simulink model "Maxpid_fermeture_geometrique_2016a"  (R2016b)
settings: Solver=VariableStepAuto  StartTime=0.0  StopTime=10.0  RelTol=1e-3
PreLoadFcn:
  | addpath('Simscape')
model workspace (MATLAB code in the model file):
  | % Simscape(TM) Multibody(TM) version: 7.0
  | 
  | % This is a model data file derived from a Simscape Multibody Import XML file using the smimport function.
  | % The data in this file sets the block parameter values in an imported Simscape Multibody model.
  | % For more information on this file, see the smimport function help page in the Simscape Multibody documentation.
  | % You can modify numerical values, but avoid any other changes to this file.
  | % Do not add code to this file. Do not edit the physical units shown in comments.
  | 
  | %%%VariableName:smiData
  | 
  | 
  | %============= RigidTransform =============%
  | 
  | %Initialize the RigidTransform structure array by filling in null values.
  | smiData.RigidTransform(52).translation = [0.0 0.0 0.0];
  | smiData.RigidTransform(52).angle = 0.0;
  | smiData.RigidTransform(52).axis = [0.0 0.0 0.0];
  | smiData.RigidTransform(52).ID = '';
  | 
  | %Translation Method - Cartesian
  | %Rotation Method - Arbitrary Axis
  | smiData.RigidTransform(1).translation = [-10.000000000000057 1.9247813558290127e-14 5.0621138792892188e-15];  % mm
  | smiData.RigidTransform(1).angle = 2.0943951023931962;  % rad
  | smiData.RigidTransform(1).axis = [-0.57735026918962473 -0.57735026918962606 0.57735026918962651];
  | smiData.RigidTransform(1).ID = 'B[vis_ass-1:-:moteur_ass-1]';
  | 
  | %Translation Method - Cartesian
  | %Rotation Method - Arbitrary Axis
  | smiData.RigidTransform(2).translation = [200.00000000000006 0.0020410288675948296 4.1211478674085811e-13];  % mm
  | smiData.RigidTransform(2).angle = 2.0943951023931966;  % rad
  | smiData.RigidTransform(2).axis = [-0.57735026918962606 -0.57735026918962618 0.57735026918962506];
  | smiData.RigidTransform(2).ID = 'F[vis_ass-1:-:moteur_ass-1]';
  | 
  | %Translation Method - Cartesian
  | %Rotation Method - Arbitrary Axis
  | smiData.RigidTransform(3).translation = [79.999999999999986 1.1487735351088687e-14 12.999999999999844];  % mm
  | smiData.RigidTransform(3).angle = 1.6411050513807407e-15;  % rad
  | smiData.RigidTransform(3).axis = [0.99999999925342131 -3.864139429547283e-05 -3.1707293661675708e-20];
  | smiData.RigidTransform(3).ID = 'B[bras_ass-1:-:ecrou_ass-1]';
  | 
  | %Translation Method - Cartesian
  | %Rotation Method - Arbitrary Axis
  | smiData.RigidTransform(4).translation = [7.6827433304060833e-14 -3.4283687000424834e-13 15.979130371550594];  % mm
  | smiData.RigidTransform(4).angle = 1.3742753698359832e-14;  % rad
  | smiData.RigidTransform(4).axis = [0.99516609511328202 -0.098206125760982824 -6.7154932536581202e-16];
  | smiData.RigidTransform(4).ID = 'F[bras_ass-1:-:ecrou_ass-1]';
  | 
  | %Translation Method - Cartesian
  | %Rotation Method - Arbitrary Axis
  | smiData.RigidTransform(5).translation = [-10.000000000000057 1.9247813558290127e-14 5.0621138792892188e-15];  % mm
  | smiData.RigidTransform(5).angle = 2.0943951023931962;  % rad
  | smiData.RigidTransform(5).axis = [-0.57735026918962473 -0.57735026918962606 0.57735026918962651];
  | smiData.RigidTransform(5).ID = 'B[vis_ass-1:-:ecrou_ass-1]';
  | 
  | %Translation Method - Cartesian
  | %Rotation Method - Arbitrary Axis
  | smiData.RigidTransform(6).translation = [-30.000729304908297 -0.50000000000034284 5.9791303715506583];  % mm
  | smiData.RigidTransform(6).angle = 2.0943951023931957;  % rad
  | smiData.RigidTransform(6).axis = [0.57735026918962562 0.57735026918962584 0.57735026918962584];
  | smiData.RigidTransform(6).ID = 'F[vis_ass-1:-:ecrou_ass-1]';
  | 
  | %Translation Method - Cartesian
  | %Rotation Method - Arbitrary Axis
  | smiData.RigidTransform(7).translation = [1.4210854715202004e-14 -1.4210854715202004e-14 -46.499999999999986];  % mm
  | smiData.RigidTransform(7).angle = 3.1401849173675503e-16;  % rad
  | smiData.RigidTransform(7).axis = [-0.70710678118654746 -0.70710678118654746 7.8504622934188746e-17];
  | smiData.RigidTransform(7).ID = 'B[bras_ass-1:-:bati_ass-1]';
  | 
  | %Translation Method - Cartesian
  | %Rotation Method - Arbitrary Axis
  | smiData.RigidTransform(8).translation = [1.4210854715202016e-14 -7.1054273576010019e-15 -48.499999999999993];  % mm
  | smiData.RigidTransform(8).angle = 4.9650683064945482e-16;  % rad
  | smiData.RigidTransform(8).axis = [-0.89442719099991519 -0.44721359549995904 9.9301366129891115e-17];
  | smiData.RigidTransform(8).ID = 'F[bras_ass-1:-:bati_ass-1]';
  | 
  | %Translation Method - Cartesian
  | %Rotation Method - Arbitrary Axis
  | smiData.RigidTransform(9).translation = [0 0 0];  % mm
  | smiData.RigidTransform(9).angle = 2.0943951023931953;  % rad
  | smiData.RigidTransform(9).axis = [-0.57735026918962584 -0.57735026918962584 -0.57735026918962584];
  | smiData.RigidTransform(9).ID = 'B[bati_ass-1:-:]';
  | 
  | %Translation Method - Cartesian
  | %Rotation Method - Arbitrary Axis
  | smiData.RigidTransform(10).translation = [0 0 0];  % mm
  | smiData.RigidTransform(10).angle = 1.5707963267948966;  % rad
  | smiData.RigidTransform(10).axis = [7.8504622934188758e-17 7.8504622934188758e-17 -1];
  | smiData.RigidTransform(10).ID = 'F[bati_ass-1:-:]';
  | 
  | %Translation Method - Cartesian
  | %Rotation Method - Arbitrary Axis
  | smiData.RigidTransform(11).translation = [-70 80 -33];  % mm
  | smiData.RigidTransform(11).angle = 0;  % rad
  | smiData.RigidTransform(11).axis = [0 0 0];
  | smiData.RigidTransform(11).ID = 'B[bati_ass-1:-:moteur_ass-1]';
  | 
  | %Translation Method - Cartesian
  | %Rotation Method - Arbitrary Axis
  | smiData.RigidTransform(12).translation = [8.5265128291212022e-14 1.7053025658242404e-13 -33.999999999999822];  % mm
  | smiData.RigidTransform(12).angle = 5.4944824200518475e-15;  % rad
  | smiData.RigidTransform(12).axis = [0.96259366809221403 -0.27094912834105328 -7.1651873630488301e-16];
  | smiData.RigidTransform(12).ID = 'F[bati_ass-1:-:moteur_ass-1]';
  | 
  | %Translation Method - Cartesian
  | %Rotation Method - Arbitrary Axis
  | smiData.RigidTransform(13).translation = [90.999999999999744 0 -33.000000000000036];  % mm
  | smiData.RigidTransform(13).angle = 3.1415926535897865;  % rad
  | smiData.RigidTransform(13).axis = [-0 -1 -0];
  | smiData.RigidTransform(13).ID = 'AssemblyGround[bras_ass-1:VisChcM4-2]';
  | 
  | %Translation Method - Cartesian
  | %Rotation Method - Arbitrary Axis
  | smiData.RigidTransform(14).translation = [79.999999999999346 8.4654505627668196e-13 -19.999999999997431];  % mm
  | smiData.RigidTransform(14).angle = 0.092778004913466591;  % rad
  | smiData.RigidTransform(14).axis = [3.4812448211815589e-13 -1.4459260087237306e-14 -1];
  | smiData.RigidTransform(14).ID = 'AssemblyGround[bras_ass-1:BagueIna12-1]';
  | 
  | %Translation Method - Cartesian
  | %Rotation Method - Arbitrary Axis
  | smiData.RigidTransform(15).translation = [79.999999999999986 0 19.999999999999844];  % mm
  | smiData.RigidTransform(15).angle = 3.1415926535897918;  % rad
  | smiData.RigidTransform(15).axis = [-0.99892422316352036 0.046372366525306442 3.8019289262458494e-17];
  | smiData.RigidTransform(15).ID = 'AssemblyGround[bras_ass-1:BagueIna12-2]';
  | 
  | %Translation Method - Cartesian
  | %Rotation Method - Arbitrary Axis
  | smiData.RigidTransform(16).translation = [0 0 47.499999999999972];  % mm
  | smiData.RigidTransform(16).angle = 2.0943951023931953;  % rad
  | smiData.RigidTransform(16).axis = [0.57735026918962573 -0.57735026918962573 0.57735026918962584];
  | smiData.RigidTransform(16).ID = 'AssemblyGround[bras_ass-1:AxeBras-1]';
  | 
  | %Translation Method - Cartesian
  | %Rotation Method - Arbitrary Axis
  | smiData.RigidTransform(17).translation = [100.50000000000018 121.50000000000016 27.999999999999993];  % mm
  | smiData.RigidTransform(17).angle = 1.5707963267948981;  % rad
  | smiData.RigidTransform(17).axis = [-0 -0 -1];
  | smiData.RigidTransform(17).ID = 'AssemblyGround[bras_ass-1:Bras-1]';
  | 
  | %Translation Method - Cartesian
  | %Rotation Method - Arbitrary Axis
  | smiData.RigidTransform(18).translation = [294.00000000000006 0 0];  % mm
  | smiData.RigidTransform(18).angle = 1.5707963267948966;  % rad
  | smiData.RigidTransform(18).axis = [0 0 -1];
  | smiData.RigidTransform(18).ID = 'AssemblyGround[bras_ass-1:Poids-3]';
  | 
  | %Translation Method - Cartesian
  | %Rotation Method - Arbitrary Axis
  | smiData.RigidTransform(19).translation = [282 0 0];  % mm
  | smiData.RigidTransform(19).angle = 1.5707963267948966;  % rad
  | smiData.RigidTransform(19).axis = [0 0 -1];
  | smiData.RigidTransform(19).ID = 'AssemblyGround[bras_ass-1:Poids-1]';
  | 
  | %Translation Method - Cartesian
  | %Rotation Method - Arbitrary Axis
  | smiData.RigidTransform(20).translation = [252.00000000000011 0 0];  % mm
  | smiData.RigidTransform(20).angle = 1.5744482311252364;  % rad
  | smiData.RigidTransform(20).axis = [-0.060320878582140823 -0.060320878582140816 -0.99635474767482157];
  | smiData.RigidTransform(20).ID = 'AssemblyGround[bras_ass-1:EcrouSerragePoids-2]';
  | 
  | %Translation Method - Cartesian
  | %Rotation Method - Arbitrary Axis
  | smiData.RigidTransform(21).translation = [91.000000000000028 0 32.999999999999993];  % mm
  | smiData.RigidTransform(21).angle = 0;  % rad
  | smiData.RigidTransform(21).axis = [0 0 0];
  | smiData.RigidTransform(21).ID = 'AssemblyGround[bras_ass-1:VisChcM4-1]';
  | 
  | %Translation Method - Cartesian
  | %Rotation Method - Arbitrary Axis
  | smiData.RigidTransform(22).translation = [80.000000000000028 0 29.999999999999982];  % mm
  | smiData.RigidTransform(22).angle = 3.1415926535897931;  % rad
  | smiData.RigidTransform(22).axis = [-0.70710678118654791 -0.70710678118654713 -3.9695354913923758e-17];
  | smiData.RigidTransform(22).ID = 'AssemblyGround[bras_ass-1:AxeArticulation-2]';
  | 
  | %Translation Method - Cartesian
  | %Rotation Method - Arbitrary Axis
  | smiData.RigidTransform(23).translation = [80.000000000000014 0 -29.999999999999989];  % mm
  | smiData.RigidTransform(23).angle = 1.5707963267948977;  % rad
  | smiData.RigidTransform(23).axis = [-0 -0 -1];
  | smiData.RigidTransform(23).ID = 'AssemblyGround[bras_ass-1:AxeArticulation-1]';
  | 
  | %Translation Method - Cartesian
  | %Rotation Method - Arbitrary Axis
  | smiData.RigidTransform(24).translation = [258.00000000000006 0 0];  % mm
  | smiData.RigidTransform(24).angle = 1.5708826466989811;  % rad
  | smiData.RigidTransform(24).axis = [-0.009290449585176894 -0.0092904495851768906 -0.999913683821264];
  | smiData.RigidTransform(24).ID = 'AssemblyGround[bras_ass-1:EcrouSerragePoids-1]';
  | 
  | %Translation Method - Cartesian
  | %Rotation Method - Arbitrary Axis
  | smiData.RigidTransform(25).translation = [237.00000000000009 3.4197923590601689 2.3580168307901075];  % mm
  | smiData.RigidTransform(25).angle = 2.718034541017071;  % rad
  | smiData.RigidTransform(25).axis = [-0.69056994469318977 -0.69056994469318989 -0.21500303014815719];
  | smiData.RigidTransform(25).ID = 'AssemblyGround[bras_ass-1:AxePoids-1]';
  | 
  | %Translation Method - Cartesian
  | %Rotation Method - Arbitrary Axis
  | smiData.RigidTransform(26).translation = [294.00000000000011 0 0];  % mm
  | smiData.RigidTransform(26).angle = 1.5987068466520886;  % rad
  | smiData.RigidTransform(26).axis = [0.16477027986751258 -0.16477027986751264 0.97247185550264792];
  | smiData.RigidTransform(26).ID = 'AssemblyGround[bras_ass-1:AxeRessort-1]';
  | 
  | %Translation Method - Cartesian
  | %Rotation Method - Arbitrary Axis
  | smiData.RigidTransform(27).translation = [270 0 0];  % mm
  | smiData.RigidTransform(27).angle = 1.5707963267948966;  % rad
  | smiData.RigidTransform(27).axis = [0 0 -1];
  | smiData.RigidTransform(27).ID = 'AssemblyGround[bras_ass-1:Poids-2]';
  | 
  | %Translation Method - Cartesian
  | %Rotation Method - Arbitrary Axis
  | smiData.RigidTransform(28).translation = [-200.00000000000011 0 0];  % mm
  | smiData.RigidTransform(28).angle = 1.6033476988916029;  % rad
  | smiData.RigidTransform(28).axis = [-0.17753814395804177 0.17753814395804177 0.96796715588901427];
  | smiData.RigidTransform(28).ID = 'AssemblyGround[vis_ass-1:EcrouM6-1]';
  | 
  | %Translation Method - Cartesian
  | %Rotation Method - Arbitrary Axis
  | smiData.RigidTransform(29).translation = [-176.00000000000009 0 0];  % mm
  | smiData.RigidTransform(29).angle = 0.51434614493842068;  % rad
  | smiData.RigidTransform(29).axis = [1 0 2.3568855398281085e-16];
  | smiData.RigidTransform(29).ID = 'AssemblyGround[vis_ass-1:VisBille-1]';
  | 
  | %Translation Method - Cartesian
  | %Rotation Method - Arbitrary Axis
  | smiData.RigidTransform(30).translation = [-10.000000000000009 0 0];  % mm
  | smiData.RigidTransform(30).angle = 0.94247779607696236;  % rad
  | smiData.RigidTransform(30).axis = [1 1.9209682992159078e-15 1.5599933518283066e-15];
  | smiData.RigidTransform(30).ID = 'AssemblyGround[vis_ass-1:RondelleVisBille-1]';
  | 
  | %Translation Method - Cartesian
  | %Rotation Method - Arbitrary Axis
  | smiData.RigidTransform(31).translation = [-207.00000000000014 0 0];  % mm
  | smiData.RigidTransform(31).angle = 1.2080018604776608;  % rad
  | smiData.RigidTransform(31).axis = [1 -8.9064014692544017e-17 0];
  | smiData.RigidTransform(31).ID = 'AssemblyGround[vis_ass-1:Accouplement-1]';
  | 
  | %Translation Method - Cartesian
  | %Rotation Method - Arbitrary Axis
  | smiData.RigidTransform(32).translation = [-195.00000000000017 0 0];  % mm
  | smiData.RigidTransform(32).angle = 2.8566332216390737;  % rad
  | smiData.RigidTransform(32).axis = [-0.69979339697627563 -0.14345174483710449 0.69979339697627541];
  | smiData.RigidTransform(32).ID = 'AssemblyGround[vis_ass-1:RondelleM6-1]';
  | 
  | %Translation Method - Cartesian
  | %Rotation Method - Arbitrary Axis
  | smiData.RigidTransform(33).translation = [-249.00000000000011 0 0];  % mm
  | smiData.RigidTransform(33).angle = 0.61326057885890328;  % rad
  | smiData.RigidTransform(33).axis = [1 -4.9895816407432893e-17 -5.3048086412437212e-16];
  | smiData.RigidTransform(33).ID = 'AssemblyGround[vis_ass-1:RotorMoteur-1]';
  | 
  | %Translation Method - Cartesian
  | %Rotation Method - Arbitrary Axis
  | smiData.RigidTransform(34).translation = [-179.00000000000006 0 0];  % mm
  | smiData.RigidTransform(34).angle = 0.072273946411088433;  % rad
  | smiData.RigidTransform(34).axis = [1 0 0];
  | smiData.RigidTransform(34).ID = 'AssemblyGround[vis_ass-1:BagueVisBille-1]';
  | 
  | %Translation Method - Cartesian
  | %Rotation Method - Arbitrary Axis
  | smiData.RigidTransform(35).translation = [-3.0000000000000444 0 0];  % mm
  | smiData.RigidTransform(35).angle = 0.82843866056758242;  % rad
  | smiData.RigidTransform(35).axis = [1 -1.1299952875043414e-16 7.5333019166956099e-17];
  | smiData.RigidTransform(35).ID = 'AssemblyGround[vis_ass-1:VisFhcM6-1]';
  | 
  | %Translation Method - Cartesian
  | %Rotation Method - Arbitrary Axis
  | smiData.RigidTransform(36).translation = [-193.00000000000011 0 0];  % mm
  | smiData.RigidTransform(36).angle = 1.136496024515387;  % rad
  | smiData.RigidTransform(36).axis = [-1 -1.1885914893422454e-16 1.223838459411135e-16];
  | smiData.RigidTransform(36).ID = 'AssemblyGround[vis_ass-1:BagueIntRoulement-1]';
  | 
  | %Translation Method - Cartesian
  | %Rotation Method - Arbitrary Axis
  | smiData.RigidTransform(37).translation = [-30 0.0020410288673958221 -21.499999999999613];  % mm
  | smiData.RigidTransform(37).angle = 1.6664335535985522;  % rad
  | smiData.RigidTransform(37).axis = [-0.29524180884432899 -0.90866085456602452 0.29524180884432827];
  | smiData.RigidTransform(37).ID = 'AssemblyGround[moteur_ass-1:VisChcM4-2]';
  | 
  | %Translation Method - Cartesian
  | %Rotation Method - Arbitrary Axis
  | smiData.RigidTransform(38).translation = [19.999999999999989 0.0020410288674443944 0];  % mm
  | smiData.RigidTransform(38).angle = 0.62831853071796473;  % rad
  | smiData.RigidTransform(38).axis = [-1 -2.8889459081957584e-15 -1.127557849593959e-15];
  | smiData.RigidTransform(38).ID = 'AssemblyGround[moteur_ass-1:SupprotVisBille-1]';
  | 
  | %Translation Method - Cartesian
  | %Rotation Method - Arbitrary Axis
  | smiData.RigidTransform(39).translation = [20.000000000000018 0.0020410288674374555 0];  % mm
  | smiData.RigidTransform(39).angle = 0.65731557306984645;  % rad
  | smiData.RigidTransform(39).axis = [1 -2.9269271194518664e-15 6.3474248646130781e-16];
  | smiData.RigidTransform(39).ID = 'AssemblyGround[moteur_ass-1:BagueExtRoulement-1]';
  | 
  | %Translation Method - Cartesian
  | %Rotation Method - Arbitrary Axis
  | smiData.RigidTransform(40).translation = [34.000000000000014 0.0020410288674374555 0];  % mm
  | smiData.RigidTransform(40).angle = 0.032120796998705951;  % rad
  | smiData.RigidTransform(40).axis = [1 0 0];
  | smiData.RigidTransform(40).ID = 'AssemblyGround[moteur_ass-1:EcrouSupportVisBille-1]';
  | 
  | %Translation Method - Cartesian
  | %Rotation Method - Arbitrary Axis
  | smiData.RigidTransform(41).translation = [-30.000000000000028 0.0020410288675068444 21.499999999999595];  % mm
  | smiData.RigidTransform(41).angle = 1.6664335535985522;  % rad
  | smiData.RigidTransform(41).axis = [-0.29524180884432899 -0.90866085456602452 0.29524180884432827];
  | smiData.RigidTransform(41).ID = 'AssemblyGround[moteur_ass-1:VisChcM4-1]';
  | 
  | %Translation Method - Cartesian
  | %Rotation Method - Arbitrary Axis
  | smiData.RigidTransform(42).translation = [-26.999999999999996 0.0020410288674513333 0];  % mm
  | smiData.RigidTransform(42).angle = 2.1991148575128614;  % rad
  | smiData.RigidTransform(42).axis = [-1 -4.8071886820195462e-16 -9.4749987733508383e-16];
  | smiData.RigidTransform(42).ID = 'AssemblyGround[moteur_ass-1:BrideMoteur-1]';
  | 
  | %Translation Method - Cartesian
  | %Rotation Method - Arbitrary Axis
  | smiData.RigidTransform(43).translation = [-31 0.0020410288674513333 0];  % mm
  | smiData.RigidTransform(43).angle = 0.050793545886475028;  % rad
  | smiData.RigidTransform(43).axis = [-1 -3.7517109526216934e-14 -1.4996924802690354e-15];
  | smiData.RigidTransform(43).ID = 'AssemblyGround[moteur_ass-1:StatorMoteur-1]';
  | 
  | %Translation Method - Cartesian
  | %Rotation Method - Arbitrary Axis
  | smiData.RigidTransform(44).translation = [-70.000000000000284 68.999999999999972 -35.999999999999467];  % mm
  | smiData.RigidTransform(44).angle = 3.1415926535897865;  % rad
  | smiData.RigidTransform(44).axis = [-0 -1 -0];
  | smiData.RigidTransform(44).ID = 'AssemblyGround[bati_ass-1:VisChcM4-2]';
  | 
  | %Translation Method - Cartesian
  | %Rotation Method - Arbitrary Axis
  | smiData.RigidTransform(45).translation = [0 0 46.000000000000085];  % mm
  | smiData.RigidTransform(45).angle = 3.1415926535897865;  % rad
  | smiData.RigidTransform(45).axis = [-1 -0 -0];
  | smiData.RigidTransform(45).ID = 'AssemblyGround[bati_ass-1:BagueIna30-2]';
  | 
  | %Translation Method - Cartesian
  | %Rotation Method - Arbitrary Axis
  | smiData.RigidTransform(46).translation = [0 0 -46];  % mm
  | smiData.RigidTransform(46).angle = 0;  % rad
  | smiData.RigidTransform(46).axis = [0 0 0];
  | smiData.RigidTransform(46).ID = 'AssemblyGround[bati_ass-1:BagueIna30-1]';
  | 
  | %Translation Method - Cartesian
  | %Rotation Method - Arbitrary Axis
  | smiData.RigidTransform(47).translation = [-69.999999999999986 79.999999999999972 33];  % mm
  | smiData.RigidTransform(47).angle = 3.1415926535897931;  % rad
  | smiData.RigidTransform(47).axis = [-1 -0 -0];
  | smiData.RigidTransform(47).ID = 'AssemblyGround[bati_ass-1:AxeArticulation-1]';
  | 
  | %Translation Method - Cartesian
  | %Rotation Method - Arbitrary Axis
  | smiData.RigidTransform(48).translation = [-70 80 -33];  % mm
  | smiData.RigidTransform(48).angle = 3.1415926535897931;  % rad
  | smiData.RigidTransform(48).axis = [0 0 1];
  | smiData.RigidTransform(48).ID = 'AssemblyGround[bati_ass-1:AxeArticulation-2]';
  | 
  | %Translation Method - Cartesian
  | %Rotation Method - Arbitrary Axis
  | smiData.RigidTransform(49).translation = [0 0 0];  % mm
  | smiData.RigidTransform(49).angle = 0;  % rad
  | smiData.RigidTransform(49).axis = [0 0 0];
  | smiData.RigidTransform(49).ID = 'AssemblyGround[bati_ass-1:Chaise-1]';
  | 
  | %Translation Method - Cartesian
  | %Rotation Method - Arbitrary Axis
  | smiData.RigidTransform(50).translation = [-70.000000000000014 69 36.000000000000007];  % mm
  | smiData.RigidTransform(50).angle = 0;  % rad
  | smiData.RigidTransform(50).axis = [0 0 0];
  | smiData.RigidTransform(50).ID = 'AssemblyGround[bati_ass-1:VisChcM4-1]';
  | 
  | %Translation Method - Cartesian
  | %Rotation Method - Arbitrary Axis
  | smiData.RigidTransform(51).translation = [40.125000000000036 16.792738254764792 -6.5847793962006174];  % mm
  | smiData.RigidTransform(51).angle = 0.62831853071794164;  % rad
  | smiData.RigidTransform(51).axis = [-1 0 0];
  | smiData.RigidTransform(51).ID = 'AssemblyGround[ecrou_ass-1:SupportEcrouBille-1]';
  | 
  | %Translation Method - Cartesian
  | %Rotation Method - Arbitrary Axis
  | smiData.RigidTransform(52).translation = [7.0000000000000338 -0.49999999999993106 5.9791303715507071];  % mm
  | smiData.RigidTransform(52).angle = 1.9713451234477288;  % rad
  | smiData.RigidTransform(52).axis = [0.52965656527971039 0.66251629845023408 0.52965656527971061];
  | smiData.RigidTransform(52).ID = 'AssemblyGround[ecrou_ass-1:EcrouBille-1]';
  | 
  | 
  | %============= Solid =============%
  | %Center of Mass (CoM) %Moments of Inertia (MoI) %Product of Inertia (PoI)
  | 
  | %Initialize the Solid structure array by filling in null values.
  | smiData.Solid(27).mass = 0.0;
  | smiData.Solid(27).CoM = [0.0 0.0 0.0];
  | smiData.Solid(27).MoI = [0.0 0.0 0.0];
  | smiData.Solid(27).PoI = [0.0 0.0 0.0];
  | smiData.Solid(27).color = [0.0 0.0 0.0];
  | smiData.Solid(27).opacity = 0.0;
  | smiData.Solid(27).ID = '';
  | 
  | %Inertia Type - Custom
  | %Visual Properties - Simple
  | smiData.Solid(1).mass = 1.913087125687861e-14;  % kg
  | smiData.Solid(1).CoM = [0.00017482716988745047 3.2099175360591674e-05 -1.3211998133732603];  % mm
  | smiData.Solid(1).MoI = [0 0 0];  % kg*mm^2
  | smiData.Solid(1).PoI = [0 0 0];  % kg*mm^2
  | smiData.Solid(1).color = [0.792156862745098 0.81960784313725488 0.93333333333333335];
  | smiData.Solid(1).opacity = 1;
  | smiData.Solid(1).ID = 'VisChcM4*:*Defaut';
  | 
  | %Inertia Type - Custom
  | %Visual Properties - Simple
  | smiData.Solid(2).mass = 4.8694686130641791e-14;  % kg
  | smiData.Solid(2).CoM = [0 0 1.848387096774194];  % mm
  | smiData.Solid(2).MoI = [0 0 0];  % kg*mm^2
  | smiData.Solid(2).PoI = [0 0 0];  % kg*mm^2
  | smiData.Solid(2).color = [1 0 0];
  | smiData.Solid(2).opacity = 1;
  | smiData.Solid(2).ID = 'BagueIna12*:*Defaut';
  | 
  | %Inertia Type - Custom
  | %Visual Properties - Simple
  | smiData.Solid(3).mass = 6.5992676097002718e-12;  % kg
  | smiData.Solid(3).CoM = [-48.219059130186579 0 0];  % mm
  | smiData.Solid(3).MoI = [7.4534196241053467e-10 5.1914505440532212e-09 5.1839580222850838e-09];  % kg*mm^2
  | smiData.Solid(3).PoI = [0 0 0];  % kg*mm^2
  | smiData.Solid(3).color = [1 0 0];
  | smiData.Solid(3).opacity = 1;
  | smiData.Solid(3).ID = 'AxeBras*:*Defaut';
  | 
  | %Inertia Type - Custom
  | %Visual Properties - Simple
  | smiData.Solid(4).mass = 1.1966905700493424e-11;  % kg
  | smiData.Solid(4).CoM = [121.52268202090545 -4.969129514901149 -27.999999999999556];  % mm
  | smiData.Solid(4).MoI = [7.7814080987725223e-08 6.582300775495296e-09 7.3498007295449486e-08];  % kg*mm^2
  | smiData.Solid(4).PoI = [0 0 0];  % kg*mm^2
  | smiData.Solid(4).color = [1 0 0];
  | smiData.Solid(4).opacity = 1;
  | smiData.Solid(4).ID = 'Bras*:*Defaut';
  | 
  | %Inertia Type - Custom
  | %Visual Properties - Simple
  | smiData.Solid(5).mass = 0.64789884834471512;  % kg
  | smiData.Solid(5).CoM = [-2.0536539050800404 -5.9999999999999627 0];  % mm
  | smiData.Solid(5).MoI = [448.87025526927192 835.42692079456913 402.10623788557024];  % kg*mm^2
  | smiData.Solid(5).PoI = [0 0 0];  % kg*mm^2
  | smiData.Solid(5).color = [1 0 0];
  | smiData.Solid(5).opacity = 1;
  | smiData.Solid(5).ID = 'Poids*:*Defaut';
  | 
  | %Inertia Type - Custom
  | %Visual Properties - Simple
  | smiData.Solid(6).mass = 1.1915826288096166e-13;  % kg
  | smiData.Solid(6).CoM = [3.6591475952249857e-05 -2.9997024398795644 2.6109734489883295e-05];  % mm
  | smiData.Solid(6).MoI = [0 0 0];  % kg*mm^2
  | smiData.Solid(6).PoI = [0 0 0];  % kg*mm^2
  | smiData.Solid(6).color = [1 0 0];
  | smiData.Solid(6).opacity = 1;
  | smiData.Solid(6).ID = 'EcrouSerragePoids*:*Defaut';
  | 
  | %Inertia Type - Custom
  | %Visual Properties - Simple
  | smiData.Solid(7).mass = 3.6367861956118845e-13;  % kg
  | smiData.Solid(7).CoM = [0 -0.11402656300615598 2.1307319223985894];  % mm
  | smiData.Solid(7).MoI = [0 0 0];  % kg*mm^2
  | smiData.Solid(7).PoI = [0 0 0];  % kg*mm^2
  | smiData.Solid(7).color = [0.792156862745098 0.81960784313725488 0.93333333333333335];
  | smiData.Solid(7).opacity = 1;
  | smiData.Solid(7).ID = 'AxeArticulation*:*Defaut';
  | 
  | %Inertia Type - Custom
  | %Visual Properties - Simple
  | smiData.Solid(8).mass = 1.2840039937491999e-12;  % kg
  | smiData.Solid(8).CoM = [-4.1541055520205505 9.4534863101010309 -2.6439442480407891e-06];  % mm
  | smiData.Solid(8).MoI = [1.2381504618383058e-09 0 1.238157782687606e-09];  % kg*mm^2
  | smiData.Solid(8).PoI = [0 0 0];  % kg*mm^2
  | smiData.Solid(8).color = [1 0 0];
  | smiData.Solid(8).opacity = 1;
  | smiData.Solid(8).ID = 'AxePoids*:*Defaut';
  | 
  | %Inertia Type - Custom
  | %Visual Properties - Simple
  | smiData.Solid(9).mass = 3.3431781821951382e-13;  % kg
  | smiData.Solid(9).CoM = [0 -8.3913860610806577 0];  % mm
  | smiData.Solid(9).MoI = [0 0 0];  % kg*mm^2
  | smiData.Solid(9).PoI = [0 0 0];  % kg*mm^2
  | smiData.Solid(9).color = [1 0 0];
  | smiData.Solid(9).opacity = 1;
  | smiData.Solid(9).ID = 'AxeRessort*:*Defaut';
  | 
  | %Inertia Type - Custom
  | %Visual Properties - Simple
  | smiData.Solid(10).mass = 3.2436540679646126e-14;  % kg
  | smiData.Solid(10).CoM = [6.6017426300604492e-05 -2.5001780719836924 0.00011392574116365407];  % mm
  | smiData.Solid(10).MoI = [0 0 0];  % kg*mm^2
  | smiData.Solid(10).PoI = [0 0 0];  % kg*mm^2
  | smiData.Solid(10).color = [0.75294117647058822 1 0.75294117647058822];
  | smiData.Solid(10).opacity = 1;
  | smiData.Solid(10).ID = 'EcrouM6*:*Defaut';
  | 
  | %Inertia Type - Custom
  | %Visual Properties - Simple
  | smiData.Solid(11).mass = 1.9275110826406196e-12;  % kg
  | smiData.Solid(11).CoM = [75.753758887885439 0 0];  % mm
  | smiData.Solid(11).MoI = [0 4.9885760188161509e-09 4.9885760188161509e-09];  % kg*mm^2
  | smiData.Solid(11).PoI = [0 0 0];  % kg*mm^2
  | smiData.Solid(11).color = [0.75294117647058822 1 0.75294117647058822];
  | smiData.Solid(11).opacity = 1;
  | smiData.Solid(11).ID = 'VisBille*:*Defaut';
  | 
  | %Inertia Type - Custom
  | %Visual Properties - Simple
  | smiData.Solid(12).mass = 1.2036446851756366e-12;  % kg
  | smiData.Solid(12).CoM = [4.9618277776521449 0.0099812415306071399 -0.013780904347995832];  % mm
  | smiData.Solid(12).MoI = [0 0 0];  % kg*mm^2
  | smiData.Solid(12).PoI = [0 0 0];  % kg*mm^2
  | smiData.Solid(12).color = [0.75294117647058822 1 0.75294117647058822];
  | smiData.Solid(12).opacity = 1;
  | smiData.Solid(12).ID = 'RondelleVisBille*:*Defaut';
  | 
  | %Inertia Type - Custom
  | %Visual Properties - Simple
  | smiData.Solid(13).mass = 5.6096059033133564e-13;  % kg
  | smiData.Solid(13).CoM = [-10.914959484771275 -0.0013517034619366178 0.0015391063193635405];  % mm
  | smiData.Solid(13).MoI = [0 0 0];  % kg*mm^2
  | smiData.Solid(13).PoI = [0 0 0];  % kg*mm^2
  | smiData.Solid(13).color = [0.75294117647058822 1 0.75294117647058822];
  | smiData.Solid(13).opacity = 1;
  | smiData.Solid(13).ID = 'Accouplement*:*Defaut';
  | 
  | %Inertia Type - Custom
  | %Visual Properties - Simple
  | smiData.Solid(14).mass = 2.5132741228718347e-14;  % kg
  | smiData.Solid(14).CoM = [0 0 -1.0000000000000002];  % mm
  | smiData.Solid(14).MoI = [0 0 0];  % kg*mm^2
  | smiData.Solid(14).PoI = [0 0 0];  % kg*mm^2
  | smiData.Solid(14).color = [0.75294117647058822 1 0.75294117647058822];
  | smiData.Solid(14).opacity = 1;
  | smiData.Solid(14).ID = 'RondelleM6*:*Defaut';
  | 
  | %Inertia Type - Custom
  | %Visual Properties - Simple
  | smiData.Solid(15).mass = 1.834794829451559e-12;  % kg
  | smiData.Solid(15).CoM = [-26.298256378060618 0 0];  % mm
  | smiData.Solid(15).MoI = [0 6.3221197317200813e-10 6.3221197317200813e-10];  % kg*mm^2
  | smiData.Solid(15).PoI = [0 0 0];  % kg*mm^2
  | smiData.Solid(15).color = [0.75294117647058822 1 0.75294117647058822];
  | smiData.Solid(15).opacity = 1;
  | smiData.Solid(15).ID = 'RotorMoteur*:*Defaut';
  | 
  | %Inertia Type - Custom
  | %Visual Properties - Simple
  | smiData.Solid(16).mass = 1.0814932709982914e-13;  % kg
  | smiData.Solid(16).CoM = [-3.2639947954490749 0 0];  % mm
  | smiData.Solid(16).MoI = [0 0 0];  % kg*mm^2
  | smiData.Solid(16).PoI = [0 0 0];  % kg*mm^2
  | smiData.Solid(16).color = [0.75294117647058822 1 0.75294117647058822];
  | smiData.Solid(16).opacity = 1;
  | smiData.Solid(16).ID = 'BagueVisBille*:*Defaut';
  | 
  | %Inertia Type - Custom
  | %Visual Properties - Simple
  | smiData.Solid(17).mass = 7.9381889668023803e-14;  % kg
  | smiData.Solid(17).CoM = [-8.1180211458661269 0 0];  % mm
  | smiData.Solid(17).MoI = [0 0 0];  % kg*mm^2
  | smiData.Solid(17).PoI = [0 0 0];  % kg*mm^2
  | smiData.Solid(17).color = [0.75294117647058822 1 0.75294117647058822];
  | smiData.Solid(17).opacity = 1;
  | smiData.Solid(17).ID = 'VisFhcM6*:*Defaut';
  | 
  | %Inertia Type - Custom
  | %Visual Properties - Simple
  | smiData.Solid(18).mass = 1.9411563965617934e-13;  % kg
  | smiData.Solid(18).CoM = [6.9999999999999911 0 0];  % mm
  | smiData.Solid(18).MoI = [0 0 0];  % kg*mm^2
  | smiData.Solid(18).PoI = [0 0 0];  % kg*mm^2
  | smiData.Solid(18).color = [0.75294117647058822 1 0.75294117647058822];
  | smiData.Solid(18).opacity = 1;
  | smiData.Solid(18).ID = 'BagueIntRoulement*:*Defaut';
  | 
  | %Inertia Type - Custom
  | %Visual Properties - Simple
  | smiData.Solid(19).mass = 6.585896472779119e-12;  % kg
  | smiData.Solid(19).CoM = [-21.219204181038748 9.0724322775607289e-05 6.9647184094088368e-05];  % mm
  | smiData.Solid(19).MoI = [2.5288316413205948e-09 2.8456398698867322e-09 2.9096770221577132e-09];  % kg*mm^2
  | smiData.Solid(19).PoI = [0 0 0];  % kg*mm^2
  | smiData.Solid(19).color = [0 0 0.75294117647058822];
  | smiData.Solid(19).opacity = 1;
  | smiData.Solid(19).ID = 'SupprotVisBille*:*Defaut';
  | 
  | %Inertia Type - Custom
  | %Visual Properties - Simple
  | smiData.Solid(20).mass = 3.8510450768364094e-13;  % kg
  | smiData.Solid(20).CoM = [7.0000319510488431 -8.0599678600116995e-05 0.00011093594041884269];  % mm
  | smiData.Solid(20).MoI = [0 0 0];  % kg*mm^2
  | smiData.Solid(20).PoI = [0 0 0];  % kg*mm^2
  | smiData.Solid(20).color = [0 0 0.75294117647058822];
  | smiData.Solid(20).opacity = 1;
  | smiData.Solid(20).ID = 'BagueExtRoulement*:*Defaut';
  | 
  | %Inertia Type - Custom
  | %Visual Properties - Simple
  | smiData.Solid(21).mass = 1.0448937165840142e-12;  % kg
  | smiData.Solid(21).CoM = [-2.3331328923633019 0 0];  % mm
  | smiData.Solid(21).MoI = [0 0 0];  % kg*mm^2
  | smiData.Solid(21).PoI = [0 0 0];  % kg*mm^2
  | smiData.Solid(21).color = [0 0 0.75294117647058822];
  | smiData.Solid(21).opacity = 1;
  | smiData.Solid(21).ID = 'EcrouSupportVisBille*:*Defaut';
  | 
  | %Inertia Type - Custom
  | %Visual Properties - Simple
  | smiData.Solid(22).mass = 7.2375749754014824e-13;  % kg
  | smiData.Solid(22).CoM = [-0.75805962995788601 0 0];  % mm
  | smiData.Solid(22).MoI = [0 0 0];  % kg*mm^2
  | smiData.Solid(22).PoI = [0 0 0];  % kg*mm^2
  | smiData.Solid(22).color = [0 0 0.75294117647058822];
  | smiData.Solid(22).opacity = 1;
  | smiData.Solid(22).ID = 'BrideMoteur*:*Defaut';
  | 
  | %Inertia Type - Custom
  | %Visual Properties - Simple
  | smiData.Solid(23).mass = 4.6775958417462935e-12;  % kg
  | smiData.Solid(23).CoM = [-40.071570092516239 0 0];  % mm
  | smiData.Solid(23).MoI = [8.8878119375049008e-10 3.4005816311117484e-09 3.4005816311117484e-09];  % kg*mm^2
  | smiData.Solid(23).PoI = [0 0 0];  % kg*mm^2
  | smiData.Solid(23).color = [0 0 0.75294117647058822];
  | smiData.Solid(23).opacity = 1;
  | smiData.Solid(23).ID = 'StatorMoteur*:*Defaut';
  | 
  | %Inertia Type - Custom
  | %Visual Properties - Simple
  | smiData.Solid(24).mass = 4.1154863762026296e-13;  % kg
  | smiData.Solid(24).CoM = [0 0 5.2290076335877904];  % mm
  | smiData.Solid(24).MoI = [0 0 0];  % kg*mm^2
  | smiData.Solid(24).PoI = [0 0 0];  % kg*mm^2
  | smiData.Solid(24).color = [0.48627450980392156 0.23529411764705882 0.015686274509803921];
  | smiData.Solid(24).opacity = 1;
  | smiData.Solid(24).ID = 'BagueIna30*:*Defaut';
  | 
  | %Inertia Type - Custom
  | %Visual Properties - Simple
  | smiData.Solid(25).mass = 6.3330866132065652e-11;  % kg
  | smiData.Solid(25).CoM = [-36.098942755399101 -23.213282269439972 3.4449046384098132];  % mm
  | smiData.Solid(25).MoI = [1.2386670399484535e-07 1.3481802068058499e-07 1.5487516217435768e-07];  % kg*mm^2
  | smiData.Solid(25).PoI = [-4.9859609267308815e-09 -7.8757870903878971e-09 2.5148102725885048e-08];  % kg*mm^2
  | smiData.Solid(25).color = [0.48627450980392156 0.23529411764705882 0.015686274509803921];
  | smiData.Solid(25).opacity = 1;
  | smiData.Solid(25).ID = 'Chaise*:*Defaut';
  | 
  | %Inertia Type - Custom
  | %Visual Properties - Simple
  | smiData.Solid(26).mass = 3.5308748010096663e-12;  % kg
  | smiData.Solid(26).CoM = [-39.280847736421187 -21.405068745767821 -0.02184130779970081];  % mm
  | smiData.Solid(26).MoI = [1.1195408099582166e-09 9.4245048603839144e-10 9.9124940774151312e-10];  % kg*mm^2
  | smiData.Solid(26).PoI = [0 0 0];  % kg*mm^2
  | smiData.Solid(26).color = [1 1 0];
  | smiData.Solid(26).opacity = 1;
  | smiData.Solid(26).ID = 'SupportEcrouBille*:*Defaut';
  | 
  | %Inertia Type - Custom
  | %Visual Properties - Simple
  | smiData.Solid(27).mass = 1.2657476801313281e-12;  % kg
  | smiData.Solid(27).CoM = [0 0 -9.3548026805658964];  % mm
  | smiData.Solid(27).MoI = [0 0 0];  % kg*mm^2
  | smiData.Solid(27).PoI = [0 0 0];  % kg*mm^2
  | smiData.Solid(27).color = [1 1 0];
  | smiData.Solid(27).opacity = 1;
  | smiData.Solid(27).ID = 'EcrouBille*:*Defaut';
  | 
  | 
  | %============= Joint =============%
  | %X Revolute Primitive (Rx) %Y Revolute Primitive (Ry) %Z Revolute Primitive (Rz)
  | %X Prismatic Primitive (Px) %Y Prismatic Primitive (Py) %Z Prismatic Primitive (Pz) %Spherical Primitive (S)
  | %Constant Velocity Primitive (CV) %Lead Screw Primitive (LS)
  | %Position Target (Pos)
  | 
  | %Initialize the CylindricalJoint structure array by filling in null values.
  | smiData.CylindricalJoint(2).Rz.Pos = 0.0;
  | smiData.CylindricalJoint(2).Pz.Pos = 0.0;
  | smiData.CylindricalJoint(2).ID = '';
  | 
  | smiData.CylindricalJoint(1).Rz.Pos = 152.09534240659505;  % deg
  | smiData.CylindricalJoint(1).Pz.Pos = 0;  % mm
  | smiData.CylindricalJoint(1).ID = '[bras_ass-1:-:ecrou_ass-1]';
  | 
  | %This joint has been chosen as a cut joint. Simscape Multibody treats cut joints as algebraic constraints to solve closed kinematic loops. The imported model does not use the state target data for this joint.
  | smiData.CylindricalJoint(2).Rz.Pos = 179.99999999999883;  % deg
  | smiData.CylindricalJoint(2).Pz.Pos = 0;  % mm
  | smiData.CylindricalJoint(2).ID = '[vis_ass-1:-:ecrou_ass-1]';
  | 
  | 
  | %Initialize the RevoluteJoint structure array by filling in null values.
  | smiData.RevoluteJoint(3).Rz.Pos = 0.0;
  | smiData.RevoluteJoint(3).ID = '';
  | 
  | smiData.RevoluteJoint(1).Rz.Pos = -6.3611093629270335e-15;  % deg
  | smiData.RevoluteJoint(1).ID = '[vis_ass-1:-:moteur_ass-1]';
  | 
  | smiData.RevoluteJoint(2).Rz.Pos = -8.5477407064331984e-14;  % deg
  | smiData.RevoluteJoint(2).ID = '[bras_ass-1:-:bati_ass-1]';
  | 
  | smiData.RevoluteJoint(3).Rz.Pos = -27.904657593404853;  % deg
  | smiData.RevoluteJoint(3).ID = '[bati_ass-1:-:moteur_ass-1]';
undefined symbols (not defined in the file or in its folder): smiData, X, Y, Z
libraries: sm_lib x144, nesl_utility x4
(part 1 of 4)
settings Model: Creator=Renaud  LastModifiedBy=rcostado
settings DataIOCC: ReturnWorkspaceOutputs=on
settings OptimizationCC: LifeSpan=inf
settings DebuggingCC: SFExecutionAtInitializationDiag=none
settings SFSimCC: SimUseLocalCustomCode=on
settings RTWCC: RTWUseLocalCustomCode=on

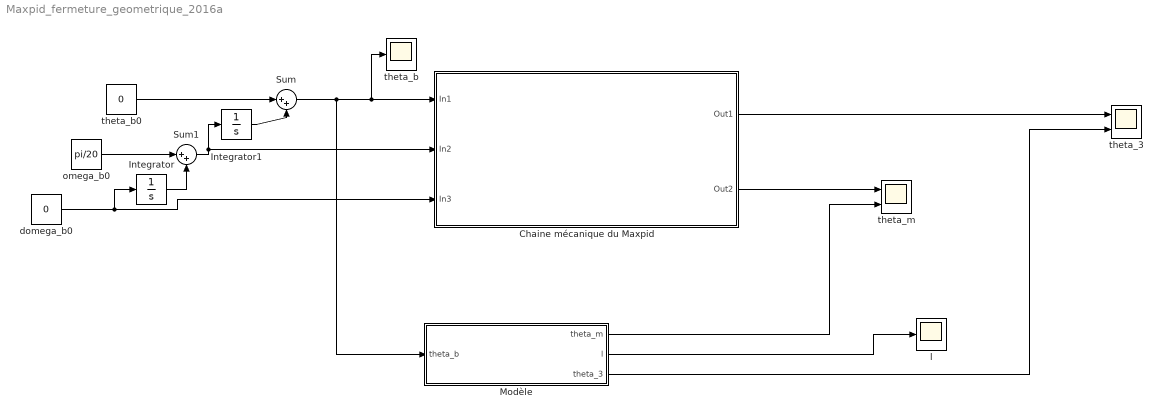
== system Maxpid_fermeture_geometrique_2016a ==
  Chaine mécanique du Maxpid : Subsystem
      mask Display: image('maxpid.png');
  Integrator : Integrator
  Integrator1 : Integrator
  Modèle : MATLAB Function  TreatAsAtomicUnit=on
  Sum : Sum  Inputs=|++
  Sum1 : Sum  Inputs=|++
  domega_b0 : Constant  Value=0
  l : Scope
  omega_b0 : Constant  Value=pi/20
  theta_3 : Scope  NumInputPorts=2
  theta_b : Scope
  theta_b0 : Constant  Value=0
  theta_m : Scope  NumInputPorts=2
  wires:
  Sum/1 -> Modèle/1(theta_b), Chaine mécanique du Maxpid/1(In1), theta_b/1
  Modèle/3(theta_3) -> theta_3/2
  Chaine mécanique du Maxpid/1(Out1) -> theta_3/1
  Modèle/2(l) -> l/1
  omega_b0/1 -> Sum1/1
  Integrator/1 -> Sum1/2
  Integrator1/1 -> Sum/2
  Sum1/1 -> Chaine mécanique du Maxpid/2(In2), Integrator1/1
  domega_b0/1 -> Chaine mécanique du Maxpid/3(In3), Integrator/1
  Chaine mécanique du Maxpid/2(Out2) -> theta_m/1
  Modèle/1(theta_m) -> theta_m/2
  theta_b0/1 -> Sum/1

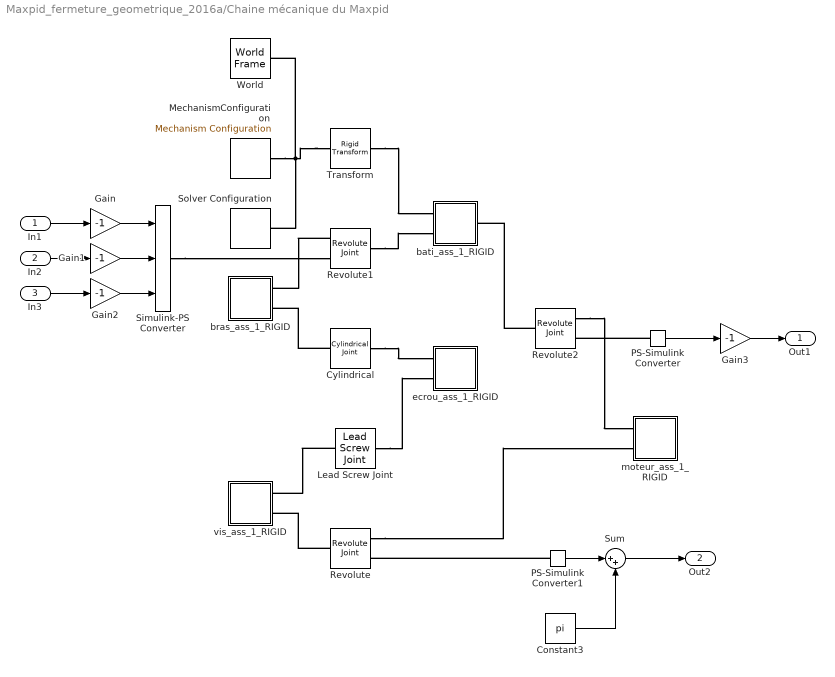
== system Maxpid_fermeture_geometrique_2016a/Chaine mécanique du Maxpid ==
  In1 : Inport
  In2 : Inport  Port=2
  In3 : Inport  Port=3
  Constant3 : Constant  Value=pi
  Cylindrical : sm_lib/Joints/Cylindrical Joint  SenseConstraintForce=off  SenseConstraintForceX=off  SenseConstraintForceY=off  SenseConstraintForceZ=off  SenseConstraintTorque=off  SenseConstraintTorqueX=off  SenseConstraintTorqueY=off  SenseConstraintTorqueZ=off  SenseTotalForce=off  SenseTotalForceX=off  SenseTotalForceY=off  SenseTotalForceZ=off  SenseTotalTorque=off  SenseTotalTorqueX=off  SenseTotalTorqueY=off  SenseTotalTorqueZ=off  CompositeWrenchDir=FollowerOnBase  CompositeWrenchFrame=BaseFrame  PzEquilibriumPosition=0  PzEquilibriumPositionUnits=m  PzSpringStiffness=0  PzSpringStiffnessUnits=N/m  PzDampingCoefficient=0  PzDampingCoefficientUnits=N/(m/s)  PzTorqueActuationMode=NoTorque  PzMotionActuationMode=ComputedMotion  PzSensePosition=off  PzSenseVelocity=off  PzSenseAcceleration=off  PzSenseTorqueForce=off  PzPositionTargetSpecify=on  PzPositionTargetPriority=Low  PzPositionTargetValue=smiData.CylindricalJoint(1).Pz.Pos  PzPositionTargetValueUnits=mm  PzVelocityTargetSpecify=off  PzVelocityTargetPriority=High  PzVelocityTargetValue=0  PzVelocityTargetValueUnits=m/s  RzEquilibriumPosition=0  RzEquilibriumPositionUnits=rad  RzSpringStiffness=0  RzSpringStiffnessUnits=N*m/rad  RzDampingCoefficient=0  RzDampingCoefficientUnits=N*m/(rad/s)  RzTorqueActuationMode=NoTorque  RzMotionActuationMode=ComputedMotion  RzSensePosition=off  RzSenseVelocity=off  RzSenseAcceleration=off  RzSenseTorqueForce=off  RzPositionTargetSpecify=on  RzPositionTargetPriority=Low  RzPositionTargetValue=smiData.CylindricalJoint(1).Rz.Pos  RzPositionTargetValueUnits=deg  RzVelocityTargetSpecify=off  RzVelocityTargetPriority=High  RzVelocityTargetValue=0  RzVelocityTargetValueUnits=deg/s
  Gain{,1..3} (4 alike) : Gain  Gain=-1
  Lead Screw Joint : sm_lib/Joints/Lead Screw Joint  SenseConstraintForce=off  SenseConstraintForceX=off  SenseConstraintForceY=off  SenseConstraintForceZ=off  SenseConstraintTorque=off  SenseConstraintTorqueX=off  SenseConstraintTorqueY=off  SenseConstraintTorqueZ=off  SenseTotalForce=off  SenseTotalForceX=off  SenseTotalForceY=off  SenseTotalForceZ=off  SenseTotalTorque=off  SenseTotalTorqueX=off  SenseTotalTorqueY=off  SenseTotalTorqueZ=off  CompositeWrenchDir=FollowerOnBase  CompositeWrenchFrame=BaseFrame  Direction=RightHand  Lead=4  LeadUnits=mm/rev  SenseRotationPosition=off  SenseRotationVelocity=off  SenseRotationAcceleration=off  SenseTranslationPosition=off  SenseTranslationVelocity=off  SenseTranslationAcceleration=off  PositionTargetSpecify=off  PositionTargetPriority=High  PositionTargetRotationBased=off  PositionTargetRotationValue=0  PositionTargetRotationValueUnits=deg  PositionTargetTranslationValue=0  PositionTargetTranslationValueUnits=m  VelocityTargetSpecify=off  VelocityTargetPriority=High  VelocityTargetRotationBased=off  VelocityTargetRotationValue=0  VelocityTargetRotationValueUnits=deg/s  VelocityTargetTranslationValue=0  VelocityTargetTranslationValueUnits=m/s
  MechanismConfiguration : sm_lib/Utilities/Mechanism Configuration  UniformGravity=Constant  GravityVector=[0 0 -9.80665]  GravityUnits=m/s^2  LinearizationDelta=0.001
  PS-Simulink Converter : nesl_utility/PS-Simulink Converter  PhysicalDomain=network_engine_domain  SubClassName=ps_output  LeftPortType=input  RightPortType=output  PseudoPeriodic=off  Frequencies=[]  Unit=rad  AffineConversion=off
  PS-Simulink Converter1 : nesl_utility/PS-Simulink Converter  PhysicalDomain=network_engine_domain  SubClassName=ps_output  LeftPortType=input  RightPortType=output  PseudoPeriodic=off  Frequencies=[]  Unit=rad  AffineConversion=off
  Revolute : sm_lib/Joints/Revolute Joint  SenseConstraintForce=off  SenseConstraintForceX=off  SenseConstraintForceY=off  SenseConstraintForceZ=off  SenseConstraintTorque=off  SenseConstraintTorqueX=off  SenseConstraintTorqueY=off  SenseConstraintTorqueZ=off  SenseTotalForce=off  SenseTotalForceX=off  SenseTotalForceY=off  SenseTotalForceZ=off  SenseTotalTorque=off  SenseTotalTorqueX=off  SenseTotalTorqueY=off  SenseTotalTorqueZ=off  CompositeWrenchDir=FollowerOnBase  CompositeWrenchFrame=BaseFrame  EquilibriumPosition=0  EquilibriumPositionUnits=rad  SpringStiffness=0  SpringStiffnessUnits=N*m/rad  DampingCoefficient=0  DampingCoefficientUnits=N*m/(rad/s)  TorqueActuationMode=NoTorque  MotionActuationMode=ComputedMotion  SensePosition=on  SenseVelocity=off  SenseAcceleration=off  SenseTorqueForce=off  PositionTargetSpecify=on  PositionTargetPriority=Low  PositionTargetValue=smiData.RevoluteJoint(1).Rz.Pos  PositionTargetValueUnits=deg  VelocityTargetSpecify=off  VelocityTargetPriority=High  VelocityTargetValue=0  VelocityTargetValueUnits=deg/s
  Revolute1 : sm_lib/Joints/Revolute Joint  SenseConstraintForce=off  SenseConstraintForceX=off  SenseConstraintForceY=off  SenseConstraintForceZ=off  SenseConstraintTorque=off  SenseConstraintTorqueX=off  SenseConstraintTorqueY=off  SenseConstraintTorqueZ=off  SenseTotalForce=off  SenseTotalForceX=off  SenseTotalForceY=off  SenseTotalForceZ=off  SenseTotalTorque=off  SenseTotalTorqueX=off  SenseTotalTorqueY=off  SenseTotalTorqueZ=off  CompositeWrenchDir=FollowerOnBase  CompositeWrenchFrame=BaseFrame  EquilibriumPosition=0  EquilibriumPositionUnits=rad  SpringStiffness=0  SpringStiffnessUnits=N*m/rad  DampingCoefficient=0  DampingCoefficientUnits=N*m/(rad/s)  TorqueActuationMode=ComputedTorque  MotionActuationMode=InputMotion  SensePosition=off  SenseVelocity=off  SenseAcceleration=off  SenseTorqueForce=off  PositionTargetSpecify=on  PositionTargetPriority=Low  PositionTargetValue=smiData.RevoluteJoint(2).Rz.Pos  PositionTargetValueUnits=deg  VelocityTargetSpecify=off  VelocityTargetPriority=High  VelocityTargetValue=0  VelocityTargetValueUnits=deg/s
  Revolute2 : sm_lib/Joints/Revolute Joint  SenseConstraintForce=off  SenseConstraintForceX=off  SenseConstraintForceY=off  SenseConstraintForceZ=off  SenseConstraintTorque=off  SenseConstraintTorqueX=off  SenseConstraintTorqueY=off  SenseConstraintTorqueZ=off  SenseTotalForce=off  SenseTotalForceX=off  SenseTotalForceY=off  SenseTotalForceZ=off  SenseTotalTorque=off  SenseTotalTorqueX=off  SenseTotalTorqueY=off  SenseTotalTorqueZ=off  CompositeWrenchDir=FollowerOnBase  CompositeWrenchFrame=BaseFrame  EquilibriumPosition=0  EquilibriumPositionUnits=rad  SpringStiffness=0  SpringStiffnessUnits=N*m/rad  DampingCoefficient=0  DampingCoefficientUnits=N*m/(rad/s)  TorqueActuationMode=NoTorque  MotionActuationMode=ComputedMotion  SensePosition=on  SenseVelocity=off  SenseAcceleration=off  SenseTorqueForce=off  PositionTargetSpecify=on  PositionTargetPriority=Low  PositionTargetValue=smiData.RevoluteJoint(3).Rz.Pos  PositionTargetValueUnits=deg  VelocityTargetSpecify=off  VelocityTargetPriority=High  VelocityTargetValue=0  VelocityTargetValueUnits=deg/s
  Simulink-PS Converter : nesl_utility/Simulink-PS Converter  PhysicalDomain=network_engine_domain  SubClassName=ps_input  LeftPortType=input  RightPortType=output  PseudoPeriodic=off  Frequencies=[]  NoiseDistribution=none  NoiseParameters=[]  Unit=1  AffineConversion=off  InputFiltering=derivs  SimscapeFilterOrder=1  InputFilterTimeConstant=0.001  UdotUserProvided=2
  Solver Configuration : nesl_utility/Solver Configuration  PhysicalDomain=network_engine_domain  SubClassName=solver  LeftPortType=input  RightPortType=generic  Accelerate=off  Tones=[]  Harmonics=[]  SimulateNoise=off  Profile=off  UseLocalSampling=off  EnableSwitchedLinearOptims=on  FrequencyDomain=off  UseCCode=off  RelTol=0.001  AbsTol=1e-06  MinStep=1e-09  ToWorkspace=off  RevertToSquareIcSolve=off  NumHomotopyIterations=100  PhasorMode=off  PhasorModeNumHarmonics=1  OverrideAbsTol=off  DoDC=off  ResidualTolerance=1e-09  UseLocalSolver=off  LocalSolverChoice=NE_BACKWARD_EULER_ADVANCER  LocalSolverSampleTime=0.001  DoFixedCost=off  MaxNonlinIter=3  MaxModeIter=2  LinearAlgebra=Sparse  DelaysMemoryBudget=1024  AutomaticFiltering=on  FilteringTimeConstant=0.001
  Sum : Sum  Inputs=|++
  Transform : sm_lib/Frames and Transforms/Rigid Transform  TranslationMethod=Cartesian  TranslationStandardOffset=0  TranslationLengthUnit=mm  TranslationStandardAxis=+Z  TranslationCartesianOffset=smiData.RigidTransform(10).translation  TranslationROffset=0  TranslationROffsetUnits=m  TranslationZOffset=0  TranslationZOffsetUnits=m  TranslationThetaOffset=0  TranslationThetaOffsetUnits=deg  RotationMethod=ArbitraryAxis  RotationAngleUnits=rad  RotationStandardAxis=+Z  RotationAngle=smiData.RigidTransform(10).angle  RotationArbitraryAxis=smiData.RigidTransform(10).axis  FollAlignAxisA=+X  BaseAlignAxisA=+Y  FollAlignAxisB=+Y  BaseAlignAxisB=+Z  RotationSequenceAxes=FollowerAxes  RotationSequence=XYX  RotationSequenceAngles=[0 0 0]  RotationSequenceAnglesUnits=deg  RotationMatrix=[1 0 0; 0 1 0; 0 0 1]
  World : sm_lib/Frames and Transforms/World Frame
  bati_ass_1_RIGID : Subsystem
  bras_ass_1_RIGID : Subsystem
  ecrou_ass_1_RIGID : Subsystem
  moteur_ass_1_RIGID : Subsystem
  vis_ass_1_RIGID : Subsystem
  Out1 : Outport
  Out2 : Outport  Port=2
  wires:
  PS-Simulink Converter/1 -> Gain3/1
  In1/1 -> Gain/1
  Constant3/1 -> Sum/2
  PS-Simulink Converter1/1 -> Sum/1
  In3/1 -> Gain2/1
  In2/1 -> Gain1/1
  Sum/1 -> Out2/1
  Gain/1 -> Simulink-PS Converter/1
  Gain1/1 -> Simulink-PS Converter/2
  Gain2/1 -> Simulink-PS Converter/3
  Gain3/1 -> Out1/1
  connections:
  PS-Simulink Converter1/LConn1 -- Revolute/RConn2
  PS-Simulink Converter/LConn1 -- Revolute2/RConn2
  Revolute2/LConn1 -- bati_ass_1_RIGID/RConn1
  Lead Screw Joint/RConn1 -- ecrou_ass_1_RIGID/LConn2
  Cylindrical/RConn1 -- ecrou_ass_1_RIGID/LConn1
  Transform/LConn1 -- MechanismConfiguration/RConn1 -- Solver Configuration/RConn1 -- World/RConn1
  Simulink-PS Converter/RConn1 -- Revolute1/LConn2
  Revolute1/RConn1 -- bati_ass_1_RIGID/LConn2
  Lead Screw Joint/LConn1 -- vis_ass_1_RIGID/RConn1
  Revolute2/RConn1 -- moteur_ass_1_RIGID/LConn1
  Revolute/RConn1 -- moteur_ass_1_RIGID/LConn2
  Revolute/LConn1 -- vis_ass_1_RIGID/RConn2
  Cylindrical/LConn1 -- bras_ass_1_RIGID/RConn2
  Revolute1/LConn1 -- bras_ass_1_RIGID/RConn1
  Transform/RConn1 -- bati_ass_1_RIGID/LConn1

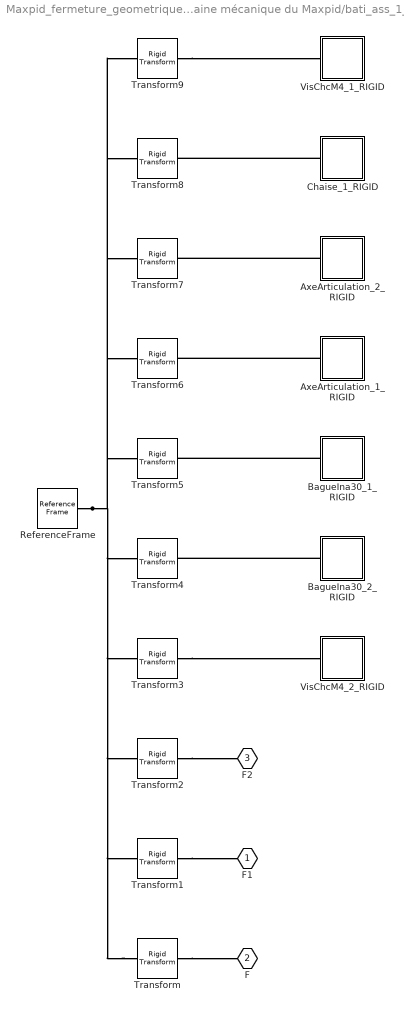
== system Maxpid_fermeture_geometrique_2016a/Chaine mécanique du Maxpid/bati_ass_1_RIGID ==
  AxeArticulation_1_RIGID : Subsystem
  AxeArticulation_2_RIGID : Subsystem
  BagueIna30_1_RIGID : Subsystem
  BagueIna30_2_RIGID : Subsystem
  Chaise_1_RIGID : Subsystem
  ReferenceFrame : sm_lib/Frames and Transforms/Reference Frame
  Transform : sm_lib/Frames and Transforms/Rigid Transform  TranslationMethod=Cartesian  TranslationStandardOffset=0  TranslationLengthUnit=mm  TranslationStandardAxis=+Z  TranslationCartesianOffset=smiData.RigidTransform(8).translation  TranslationROffset=0  TranslationROffsetUnits=m  TranslationZOffset=0  TranslationZOffsetUnits=m  TranslationThetaOffset=0  TranslationThetaOffsetUnits=deg  RotationMethod=ArbitraryAxis  RotationAngleUnits=rad  RotationStandardAxis=+Z  RotationAngle=smiData.RigidTransform(8).angle  RotationArbitraryAxis=smiData.RigidTransform(8).axis  FollAlignAxisA=+X  BaseAlignAxisA=+Y  FollAlignAxisB=+Y  BaseAlignAxisB=+Z  RotationSequenceAxes=FollowerAxes  RotationSequence=XYX  RotationSequenceAngles=[0 0 0]  RotationSequenceAnglesUnits=deg  RotationMatrix=[1 0 0; 0 1 0; 0 0 1]
  Transform1 : sm_lib/Frames and Transforms/Rigid Transform  TranslationMethod=Cartesian  TranslationStandardOffset=0  TranslationLengthUnit=mm  TranslationStandardAxis=+Z  TranslationCartesianOffset=smiData.RigidTransform(9).translation  TranslationROffset=0  TranslationROffsetUnits=m  TranslationZOffset=0  TranslationZOffsetUnits=m  TranslationThetaOffset=0  TranslationThetaOffsetUnits=deg  RotationMethod=ArbitraryAxis  RotationAngleUnits=rad  RotationStandardAxis=+Z  RotationAngle=smiData.RigidTransform(9).angle  RotationArbitraryAxis=smiData.RigidTransform(9).axis  FollAlignAxisA=+X  BaseAlignAxisA=+Y  FollAlignAxisB=+Y  BaseAlignAxisB=+Z  RotationSequenceAxes=FollowerAxes  RotationSequence=XYX  RotationSequenceAngles=[0 0 0]  RotationSequenceAnglesUnits=deg  RotationMatrix=[1 0 0; 0 1 0; 0 0 1]
  Transform2 : sm_lib/Frames and Transforms/Rigid Transform  TranslationMethod=Cartesian  TranslationStandardOffset=0  TranslationLengthUnit=mm  TranslationStandardAxis=+Z  TranslationCartesianOffset=smiData.RigidTransform(11).translation  TranslationROffset=0  TranslationROffsetUnits=m  TranslationZOffset=0  TranslationZOffsetUnits=m  TranslationThetaOffset=0  TranslationThetaOffsetUnits=deg  RotationMethod=ArbitraryAxis  RotationAngleUnits=rad  RotationStandardAxis=+Z  RotationAngle=smiData.RigidTransform(11).angle  RotationArbitraryAxis=smiData.RigidTransform(11).axis  FollAlignAxisA=+X  BaseAlignAxisA=+Y  FollAlignAxisB=+Y  BaseAlignAxisB=+Z  RotationSequenceAxes=FollowerAxes  RotationSequence=XYX  RotationSequenceAngles=[0 0 0]  RotationSequenceAnglesUnits=deg  RotationMatrix=[1 0 0; 0 1 0; 0 0 1]
  Transform3 : sm_lib/Frames and Transforms/Rigid Transform  TranslationMethod=Cartesian  TranslationStandardOffset=0  TranslationLengthUnit=mm  TranslationStandardAxis=+Z  TranslationCartesianOffset=smiData.RigidTransform(44).translation  TranslationROffset=0  TranslationROffsetUnits=m  TranslationZOffset=0  TranslationZOffsetUnits=m  TranslationThetaOffset=0  TranslationThetaOffsetUnits=deg  RotationMethod=ArbitraryAxis  RotationAngleUnits=rad  RotationStandardAxis=+Z  RotationAngle=smiData.RigidTransform(44).angle  RotationArbitraryAxis=smiData.RigidTransform(44).axis  FollAlignAxisA=+X  BaseAlignAxisA=+Y  FollAlignAxisB=+Y  BaseAlignAxisB=+Z  RotationSequenceAxes=FollowerAxes  RotationSequence=XYX  RotationSequenceAngles=[0 0 0]  RotationSequenceAnglesUnits=deg  RotationMatrix=[1 0 0; 0 1 0; 0 0 1]
  Transform4 : sm_lib/Frames and Transforms/Rigid Transform  TranslationMethod=Cartesian  TranslationStandardOffset=0  TranslationLengthUnit=mm  TranslationStandardAxis=+Z  TranslationCartesianOffset=smiData.RigidTransform(45).translation  TranslationROffset=0  TranslationROffsetUnits=m  TranslationZOffset=0  TranslationZOffsetUnits=m  TranslationThetaOffset=0  TranslationThetaOffsetUnits=deg  RotationMethod=ArbitraryAxis  RotationAngleUnits=rad  RotationStandardAxis=+Z  RotationAngle=smiData.RigidTransform(45).angle  RotationArbitraryAxis=smiData.RigidTransform(45).axis  FollAlignAxisA=+X  BaseAlignAxisA=+Y  FollAlignAxisB=+Y  BaseAlignAxisB=+Z  RotationSequenceAxes=FollowerAxes  RotationSequence=XYX  RotationSequenceAngles=[0 0 0]  RotationSequenceAnglesUnits=deg  RotationMatrix=[1 0 0; 0 1 0; 0 0 1]
  Transform5 : sm_lib/Frames and Transforms/Rigid Transform  TranslationMethod=Cartesian  TranslationStandardOffset=0  TranslationLengthUnit=mm  TranslationStandardAxis=+Z  TranslationCartesianOffset=smiData.RigidTransform(46).translation  TranslationROffset=0  TranslationROffsetUnits=m  TranslationZOffset=0  TranslationZOffsetUnits=m  TranslationThetaOffset=0  TranslationThetaOffsetUnits=deg  RotationMethod=ArbitraryAxis  RotationAngleUnits=rad  RotationStandardAxis=+Z  RotationAngle=smiData.RigidTransform(46).angle  RotationArbitraryAxis=smiData.RigidTransform(46).axis  FollAlignAxisA=+X  BaseAlignAxisA=+Y  FollAlignAxisB=+Y  BaseAlignAxisB=+Z  RotationSequenceAxes=FollowerAxes  RotationSequence=XYX  RotationSequenceAngles=[0 0 0]  RotationSequenceAnglesUnits=deg  RotationMatrix=[1 0 0; 0 1 0; 0 0 1]
  Transform6 : sm_lib/Frames and Transforms/Rigid Transform  TranslationMethod=Cartesian  TranslationStandardOffset=0  TranslationLengthUnit=mm  TranslationStandardAxis=+Z  TranslationCartesianOffset=smiData.RigidTransform(47).translation  TranslationROffset=0  TranslationROffsetUnits=m  TranslationZOffset=0  TranslationZOffsetUnits=m  TranslationThetaOffset=0  TranslationThetaOffsetUnits=deg  RotationMethod=ArbitraryAxis  RotationAngleUnits=rad  RotationStandardAxis=+Z  RotationAngle=smiData.RigidTransform(47).angle  RotationArbitraryAxis=smiData.RigidTransform(47).axis  FollAlignAxisA=+X  BaseAlignAxisA=+Y  FollAlignAxisB=+Y  BaseAlignAxisB=+Z  RotationSequenceAxes=FollowerAxes  RotationSequence=XYX  RotationSequenceAngles=[0 0 0]  RotationSequenceAnglesUnits=deg  RotationMatrix=[1 0 0; 0 1 0; 0 0 1]
  Transform7 : sm_lib/Frames and Transforms/Rigid Transform  TranslationMethod=Cartesian  TranslationStandardOffset=0  TranslationLengthUnit=mm  TranslationStandardAxis=+Z  TranslationCartesianOffset=smiData.RigidTransform(48).translation  TranslationROffset=0  TranslationROffsetUnits=m  TranslationZOffset=0  TranslationZOffsetUnits=m  TranslationThetaOffset=0  TranslationThetaOffsetUnits=deg  RotationMethod=ArbitraryAxis  RotationAngleUnits=rad  RotationStandardAxis=+Z  RotationAngle=smiData.RigidTransform(48).angle  RotationArbitraryAxis=smiData.RigidTransform(48).axis  FollAlignAxisA=+X  BaseAlignAxisA=+Y  FollAlignAxisB=+Y  BaseAlignAxisB=+Z  RotationSequenceAxes=FollowerAxes  RotationSequence=XYX  RotationSequenceAngles=[0 0 0]  RotationSequenceAnglesUnits=deg  RotationMatrix=[1 0 0; 0 1 0; 0 0 1]
  Transform8 : sm_lib/Frames and Transforms/Rigid Transform  TranslationMethod=Cartesian  TranslationStandardOffset=0  TranslationLengthUnit=mm  TranslationStandardAxis=+Z  TranslationCartesianOffset=smiData.RigidTransform(49).translation  TranslationROffset=0  TranslationROffsetUnits=m  TranslationZOffset=0  TranslationZOffsetUnits=m  TranslationThetaOffset=0  TranslationThetaOffsetUnits=deg  RotationMethod=ArbitraryAxis  RotationAngleUnits=rad  RotationStandardAxis=+Z  RotationAngle=smiData.RigidTransform(49).angle  RotationArbitraryAxis=smiData.RigidTransform(49).axis  FollAlignAxisA=+X  BaseAlignAxisA=+Y  FollAlignAxisB=+Y  BaseAlignAxisB=+Z  RotationSequenceAxes=FollowerAxes  RotationSequence=XYX  RotationSequenceAngles=[0 0 0]  RotationSequenceAnglesUnits=deg  RotationMatrix=[1 0 0; 0 1 0; 0 0 1]
  Transform9 : sm_lib/Frames and Transforms/Rigid Transform  TranslationMethod=Cartesian  TranslationStandardOffset=0  TranslationLengthUnit=mm  TranslationStandardAxis=+Z  TranslationCartesianOffset=smiData.RigidTransform(50).translation  TranslationROffset=0  TranslationROffsetUnits=m  TranslationZOffset=0  TranslationZOffsetUnits=m  TranslationThetaOffset=0  TranslationThetaOffsetUnits=deg  RotationMethod=ArbitraryAxis  RotationAngleUnits=rad  RotationStandardAxis=+Z  RotationAngle=smiData.RigidTransform(50).angle  RotationArbitraryAxis=smiData.RigidTransform(50).axis  FollAlignAxisA=+X  BaseAlignAxisA=+Y  FollAlignAxisB=+Y  BaseAlignAxisB=+Z  RotationSequenceAxes=FollowerAxes  RotationSequence=XYX  RotationSequenceAngles=[0 0 0]  RotationSequenceAnglesUnits=deg  RotationMatrix=[1 0 0; 0 1 0; 0 0 1]
  VisChcM4_1_RIGID : Subsystem
  VisChcM4_2_RIGID : Subsystem
  F1 : PMIOPort  Port=1  Side=Left
  F : PMIOPort  Port=2  Side=Left
  F2 : PMIOPort  Port=3  Side=Right
  connections:
  Transform/LConn1 -- ReferenceFrame/RConn1 -- Transform1/LConn1 -- Transform2/LConn1 -- Transform3/LConn1 -- Transform4/LConn1 -- Transform5/LConn1 -- Transform6/LConn1 -- Transform7/LConn1 -- Transform8/LConn1 -- Transform9/LConn1
  Transform/RConn1 -- F/RConn1
  Transform9/RConn1 -- VisChcM4_1_RIGID/LConn1
  Transform1/RConn1 -- F1/RConn1
  Transform2/RConn1 -- F2/RConn1
  Transform3/RConn1 -- VisChcM4_2_RIGID/LConn1
  BagueIna30_2_RIGID/LConn1 -- Transform4/RConn1
  BagueIna30_1_RIGID/LConn1 -- Transform5/RConn1
  AxeArticulation_1_RIGID/LConn1 -- Transform6/RConn1
  AxeArticulation_2_RIGID/LConn1 -- Transform7/RConn1
  Chaise_1_RIGID/LConn1 -- Transform8/RConn1
